simulink model "SCCS_FaultHandling_04"  (R2024a)
settings: Solver=ode3  StartTime=0.0  StopTime=5  FixedStep=0.01  RelTol=1e-3
settings Model: Creator=Kishore  LastModifiedBy=Kishore

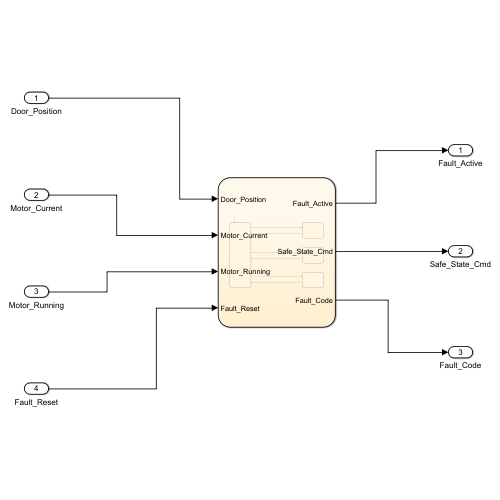
[thumbnail: Simulink's stored preview of the top-level diagram]
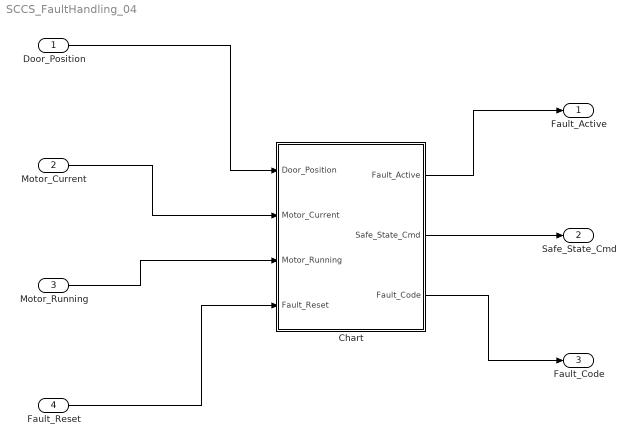
== system SCCS_FaultHandling_04 ==
  Door_Position : Inport
  Motor_Current : Inport  Port=2
  Motor_Running : Inport  Port=3
  Fault_Reset : Inport  Port=4
  Chart : Stateflow chart  TreatAsAtomicUnit=on
  Fault_Active : Outport
  Safe_State_Cmd : Outport  Port=2
  Fault_Code : Outport  Port=3
  wires:
  Door_Position/1 -> Chart/1(Door_Position)
  Motor_Current/1 -> Chart/2(Motor_Current)
  Motor_Running/1 -> Chart/3(Motor_Running)
  Fault_Reset/1 -> Chart/4(Fault_Reset)
  Chart/1(Fault_Active) -> Fault_Active/1
  Chart/2(Safe_State_Cmd) -> Safe_State_Cmd/1
  Chart/3(Fault_Code) -> Fault_Code/1

== stateflow chart SCCS_FaultHandling_04/Chart ==
  state FAULT_POSITION
    entry:
    Fault_Active = 1;
    Safe_State_Cmd = 1;
    Fault_Code = 1;
  state NORMAL
    entry:
    Fault_Active = 0;
    Safe_State_Cmd = 0;
    Fault_Code = 0;
  state FAULT_CURRENT
    entry:
    Fault_Active = 1;
    Safe_State_Cmd = 1;
    Fault_Code = 2;
  state FAULT_OVER
    entry:
    Fault_Active = 1;
    Safe_State_Cmd = 1;
    Fault_Code = 3;
  (default) -> NORMAL
  NORMAL -> FAULT_POSITION [order 1] : [Door_Position == 0 && Motor_Running == 1]
  FAULT_POSITION -> NORMAL : [Fault_Reset == 1]
  NORMAL -> FAULT_CURRENT [order 2] : [Motor_Current == 0 && Motor_Running == 1]
  FAULT_CURRENT -> NORMAL : [Fault_Reset == 1]
  NORMAL -> FAULT_OVER [order 3] : [Door_Position > 420 || Door_Position < -20]
  FAULT_OVER -> NORMAL : [Fault_Reset == 1]
  data: Door_Position input; Motor_Current input; Motor_Running input; Fault_Reset input; Fault_Active output; Safe_State_Cmd output; Fault_Code output
